simulink model "Subchart_SuperTransition"  (R2025b)
settings: Solver=FixedStepDiscrete  StartTime=0.0  StopTime=10.0  FixedStep=0.01  RelTol=1e-3
libraries: simulink x1
settings Model: Creator=soura  LastModifiedBy=soura

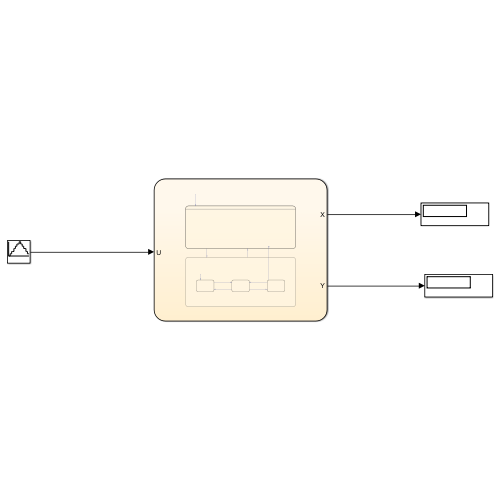
[thumbnail: Simulink's stored preview of the top-level diagram]
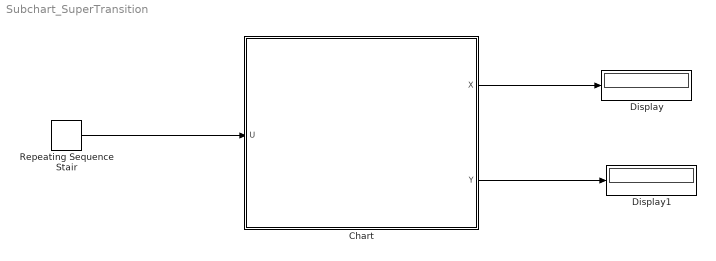
== system Subchart_SuperTransition ==
  Chart : Stateflow chart  TreatAsAtomicUnit=on
  Display : Display
  Display1 : Display
  Repeating Sequence Stair : simulink/Sources/Repeating Sequence Stair  OutValues=[0 0 1 1 2 2 3 3 4 4 5 5 6 6 5 5 4 4 3 3 2 2 1 1 ].'  tsamp=-1  OutMin=[]  OutMax=[]  OutDataTypeStr=double  OutputDataTypeScalingMode=double  OutDataType=fixdt(0,8)  ConRadixGroup=Best Precision: Vector-wise  OutScaling=2^-12
  wires:
  Repeating Sequence Stair/1 -> Chart/1(U)
  Chart/1(X) -> Display/1
  Chart/2(Y) -> Display1/1

== stateflow chart Subchart_SuperTransition/Chart ==
  state A
    state state1
      en:X=0;
    state state2
      en:X=1;
    state state3
      en:X=2;
    (default) -> state1
    state2 -> state1 [order 2] : [U==0]
    state3 -> state2 : [U==1]
    state1 -> state2 : [U==1]
    state2 -> state3 [order 1] : [U==2]
  state B
    state Low
      en:Y=0;
    state Medium
      en:Y=1;
    state High
      en:Y=2;
      du: send (E)
    (default) -> Low
    Low -> Medium : [U==4]
    High -> Medium [order 1] : [U==4]
    Medium -> Low [order 1] : [U==3]
    Medium -> High [order 2] : [U==5]
  High -> state3 [order 2] : E
  (default) -> A
  A -> B : [U>2]
  B -> A : [U<2]
  data: X output; Y output; U input
  events: E local FUNCTION_CALL_EVENT
